simulink model "Impedance_desired"  (R2022b)
settings: Solver=VariableStepAuto  StartTime=0.0  StopTime=10.0  RelTol=1e-3
values from neighbouring files (symbols this model uses):
  Kd = diag([10,10,10,1,1,1])    [parameters.m]
  Kp = diag([190,190,190,1,1,1])    [parameters.m]
  Md = diag([0.12,0.12,0.12,0,0,0])    [parameters.m]
undefined symbols (not defined in the file or in its folder): parms
libraries: robotcorelib x1
settings Model: Creator=uzair  LastModifiedBy=uzair

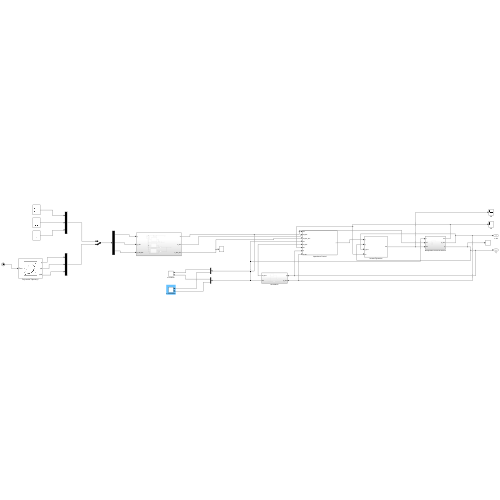
[thumbnail: Simulink's stored preview of the top-level diagram]
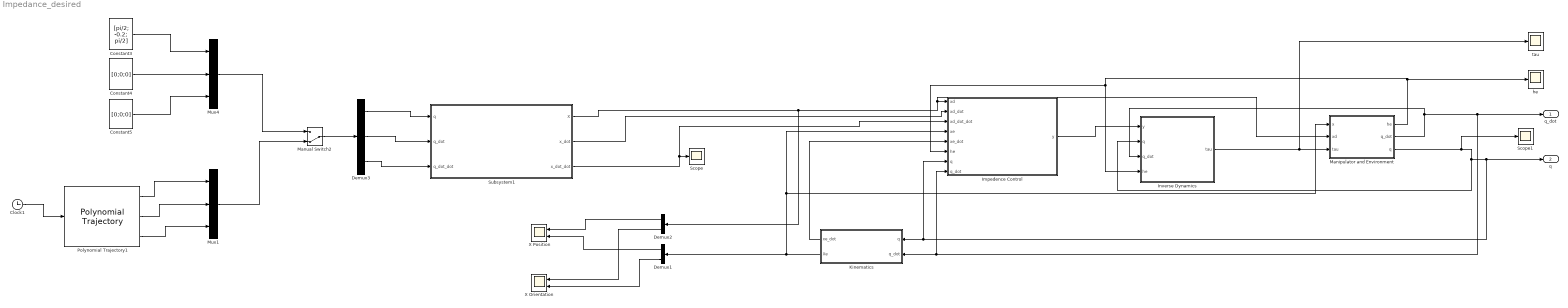
== system Impedance_desired ==
  Clock1 : Clock
  Constant3 : Constant  Value=[pi/2; -0.2; pi/2]  VectorParams1D=off
  Constant4 : Constant  Value=[0;0;0]  VectorParams1D=off
  Constant5 : Constant  Value=[0;0;0]  VectorParams1D=off
  Demux1 : Demux  Outputs=2
  Demux2 : Demux  Outputs=2
  Demux3 : Demux  Outputs=3
  Impedence Control : Subsystem
  Inverse Dynamics : Subsystem
  Kinematics : Subsystem
  Manipulator and Environment : Subsystem
  Manual Switch2 : ManualSwitch  CurrentSetting=0
  Mux1 : Mux  Inputs=3
  Mux4 : Mux  Inputs=3
  Polynomial Trajectory1 : robotcorelib/Polynomial Trajectory  WaypointSource=Internal  Waypoints=[0,0,0; 0,0,0; 0,0,0.1]  TimePoints=[ 0, 4, 9]  TimeInterval=[ 1, 4 ]  Method=Cubic Polynomial  ParameterSource=Internal  VelocityBoundaryCondition=zeros( 3,3 )  AccelerationBoundaryCondition=zeros( 3,3 )  SimulateUsing=Interpreted execution
  Scope : Scope
  Scope1 : Scope
  Subsystem1 : Subsystem
  X Orientation : Scope  NumInputPorts=2
  X Position : Scope  NumInputPorts=2
  he : Scope
  tau : Scope
  q_dot : Outport
  q : Outport  Port=2
  wires:
  Manipulator and Environment/2(q_dot) -> Inverse Dynamics/3(q_dot), Impedence Control/8(q_dot), Kinematics/2(q_dot), q_dot/1
  Manipulator and Environment/3(q) -> Scope1/1, Kinematics/1(q), Impedence Control/7(q), q/1, Inverse Dynamics/2(q)
  Inverse Dynamics/1(tau) -> tau/1, Manipulator and Environment/3(tau)
  Demux1/2 -> X Orientation/2
  Demux2/2 -> X Orientation/1
  Demux2/1 -> X Position/1
  Demux1/1 -> X Position/2
  Kinematics/2(Xe) -> Manipulator and Environment/1(x), Impedence Control/4(xe), Demux1/1
  Subsystem1/2(x_dot) -> Impedence Control/2(xd_dot)
  Subsystem1/3(x_dot_dot) -> Scope/1, Impedence Control/3(xd_dot_dot)
  Kinematics/1(xe_dot) -> Impedence Control/5(xe_dot)
  Impedence Control/1(y) -> Inverse Dynamics/1(y)
  Manipulator and Environment/1(he) -> Inverse Dynamics/4(he), Impedence Control/6(he), he/1
  Subsystem1/1(X) -> Demux2/1, Manipulator and Environment/2(xd), Impedence Control/1(xd)
  Manual Switch2/1 -> Demux3/1
  Mux4/1 -> Manual Switch2/1
  Constant4/1 -> Mux4/2
  Polynomial Trajectory1/1 -> Mux1/1
  Polynomial Trajectory1/3 -> Mux1/3
  Mux1/1 -> Manual Switch2/2
  Constant5/1 -> Mux4/3
  Demux3/1 -> Subsystem1/1(q)
  Clock1/1 -> Polynomial Trajectory1/1
  Constant3/1 -> Mux4/1
  Demux3/3 -> Subsystem1/3(q_dot_dot)
  Polynomial Trajectory1/2 -> Mux1/2
  Demux3/2 -> Subsystem1/2(q_dot)

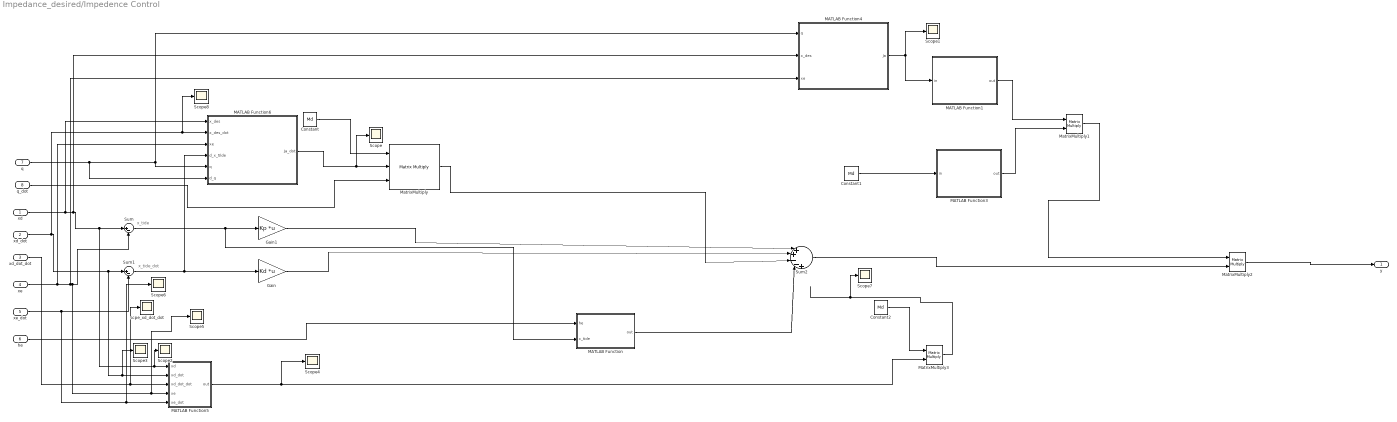
== system Impedance_desired/Impedence Control ==
  note: x_tide_dot
  note: x_tide
  xd : Inport
  xd_dot : Inport  Port=2
  xd_dot_dot : Inport  Port=3
  xe : Inport  Port=4
  xe_dot : Inport  Port=5
  he : Inport  Port=6
  q : Inport  Port=7
  q_dot : Inport  Port=8
  Constant : Constant  Value=Md  VectorParams1D=off
  Constant1 : Constant  Value=Md  VectorParams1D=off
  Constant2 : Constant  Value=Md
  Gain : Gain  Gain=Kd  Multiplication=Matrix(K*u)
  Gain1 : Gain  Gain=Kp  Multiplication=Matrix(K*u)
  MATLAB Function : MATLAB Function  TreatAsAtomicUnit=on
  MATLAB Function1 : MATLAB Function  TreatAsAtomicUnit=on
  MATLAB Function3 : MATLAB Function  TreatAsAtomicUnit=on
  MATLAB Function4 : MATLAB Function  TreatAsAtomicUnit=on
  MATLAB Function5 : MATLAB Function  TreatAsAtomicUnit=on
  MATLAB Function6 : MATLAB Function  TreatAsAtomicUnit=on
  MatrixMultiply : Product  Inputs=3  Multiplication=Matrix(*)
  MatrixMultiply1 : Product  Multiplication=Matrix(*)
  MatrixMultiply2 : Product  Multiplication=Matrix(*)
  MatrixMultiply3 : Product  Multiplication=Matrix(*)
  Scope{,1..8} (9 alike) : Scope
  Sum : Sum  Inputs=|+-
  Sum1 : Sum  Inputs=|+-
  Sum2 : Sum  Inputs=|++--+
  scpe_xd_dot_dot : Scope
  y : Outport
  wires:
  xd/1 -> MATLAB Function6/1(x_des), MATLAB Function4/2(x_des), Scope2/1, MATLAB Function5/1(xd), Sum/1
  xe/1 -> MATLAB Function6/3(xe), MATLAB Function4/3(xe), Scope5/1, MATLAB Function5/4(xe), Sum/2
  Sum/1 -> MATLAB Function/2(x_tide), Gain1/1
  xd_dot/1 -> Scope8/1, MATLAB Function6/2(x_des_dot), MATLAB Function5/2(xd_dot), Scope3/1, Sum1/1
  xe_dot/1 -> MATLAB Function5/5(xe_dot), Scope6/1, Sum1/2
  Sum1/1 -> MATLAB Function6/4(d_x_tilde), Gain/1
  Gain1/1 -> Sum2/1
  Gain/1 -> Sum2/2
  q/1 -> MATLAB Function6/6(d_q), MATLAB Function4/1(q), MATLAB Function6/5(q)
  q_dot/1 -> MatrixMultiply/3
  Constant/1 -> MatrixMultiply/1
  MATLAB Function6/1(Ja_dot) -> Scope/1, MatrixMultiply/2
  MatrixMultiply/1 -> Sum2/3
  he/1 -> MATLAB Function/1(he)
  MATLAB Function/1(out) -> Sum2/4
  MATLAB Function1/1(out) -> MatrixMultiply1/1
  MATLAB Function3/1(out) -> MatrixMultiply1/2
  MATLAB Function4/1(Ja) -> MATLAB Function1/1(in), Scope1/1
  Constant1/1 -> MATLAB Function3/1(in)
  Sum2/1 -> MatrixMultiply2/2
  MatrixMultiply1/1 -> MatrixMultiply2/1
  MatrixMultiply2/1 -> y/1
  MATLAB Function5/1(out) -> Scope4/1, MatrixMultiply3/2
  Constant2/1 -> MatrixMultiply3/1
  MatrixMultiply3/1 -> Scope7/1
  xd_dot_dot/1 -> MATLAB Function5/3(xd_dot_dot), scpe_xd_dot_dot/1

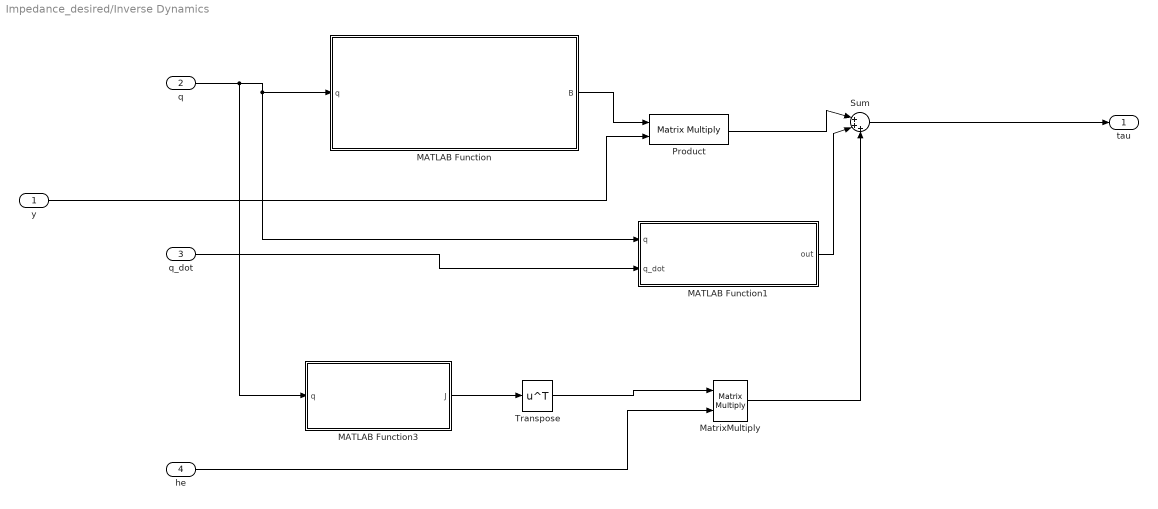
== system Impedance_desired/Inverse Dynamics ==
  y : Inport
  q : Inport  Port=2
  q_dot : Inport  Port=3
  he : Inport  Port=4
  MATLAB Function : MATLAB Function  TreatAsAtomicUnit=on
  MATLAB Function1 : MATLAB Function  TreatAsAtomicUnit=on
  MATLAB Function3 : MATLAB Function  TreatAsAtomicUnit=on
  MatrixMultiply : Product  Multiplication=Matrix(*)
  Product : Product  Multiplication=Matrix(*)
  Sum : Sum  Inputs=|+++
  Transpose : Math  Operator=transpose
  tau : Outport
  wires:
  q/1 -> MATLAB Function3/1(q), MATLAB Function1/1(q), MATLAB Function/1(q)
  MATLAB Function/1(B) -> Product/1
  y/1 -> Product/2
  q_dot/1 -> MATLAB Function1/2(q_dot)
  MATLAB Function1/1(out) -> Sum/2
  Sum/1 -> tau/1
  MATLAB Function3/1(J) -> Transpose/1
  he/1 -> MatrixMultiply/2
  Transpose/1 -> MatrixMultiply/1
  MatrixMultiply/1 -> Sum/3
  Product/1 -> Sum/1

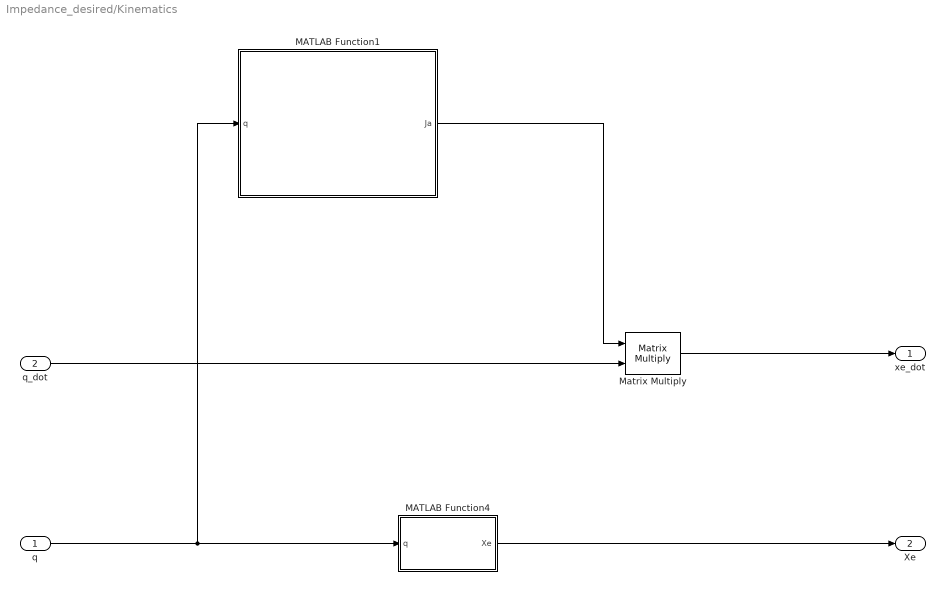
== system Impedance_desired/Kinematics ==
  q : Inport
  q_dot : Inport  Port=2
  MATLAB Function1 : MATLAB Function  TreatAsAtomicUnit=on
  MATLAB Function4 : MATLAB Function  TreatAsAtomicUnit=on
  Matrix Multiply : Product  Multiplication=Matrix(*)
  xe_dot : Outport
  Xe : Outport  Port=2
  wires:
  MATLAB Function1/1(Ja) -> Matrix Multiply/1
  q/1 -> MATLAB Function1/1(q), MATLAB Function4/1(q)
  MATLAB Function4/1(Xe) -> Xe/1
  Matrix Multiply/1 -> xe_dot/1
  q_dot/1 -> Matrix Multiply/2

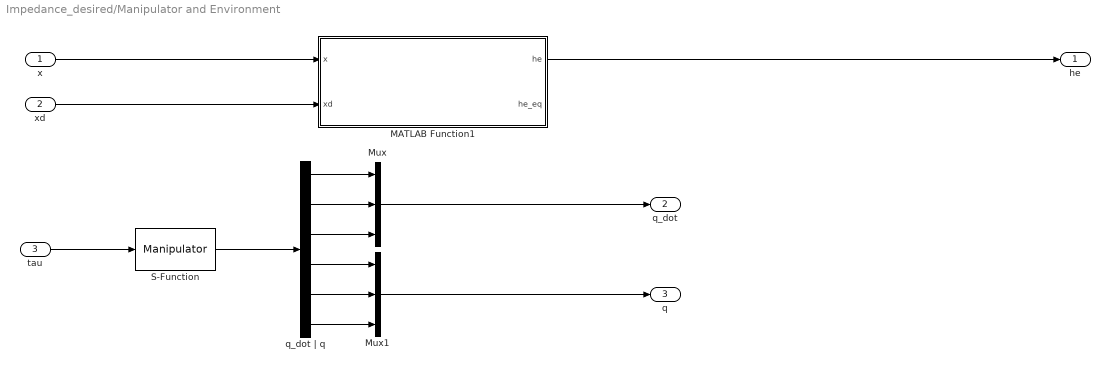
== system Impedance_desired/Manipulator and Environment ==
  x : Inport
  xd : Inport  Port=2
  tau : Inport  Port=3
  MATLAB Function1 : MATLAB Function  TreatAsAtomicUnit=on
  Mux : Mux  Inputs=3
  Mux1 : Mux  Inputs=3
  S-Function : S-Function  FunctionName=Manipulator  Parameters=params  SFunctionDeploymentMode=off  EnableBusSupport=off
  q_dot | q : Demux  Outputs=6
  he : Outport
  q_dot : Outport  Port=2
  q : Outport  Port=3
  wires:
  x/1 -> MATLAB Function1/1(x)
  xd/1 -> MATLAB Function1/2(xd)
  MATLAB Function1/1(he) -> he/1
  S-Function/1 -> q_dot | q/1
  q_dot | q/4 -> Mux1/1
  q_dot | q/1 -> Mux/1
  q_dot | q/6 -> Mux1/3
  q_dot | q/2 -> Mux/2
  q_dot | q/5 -> Mux1/2
  q_dot | q/3 -> Mux/3
  Mux/1 -> q_dot/1
  Mux1/1 -> q/1
  tau/1 -> S-Function/1

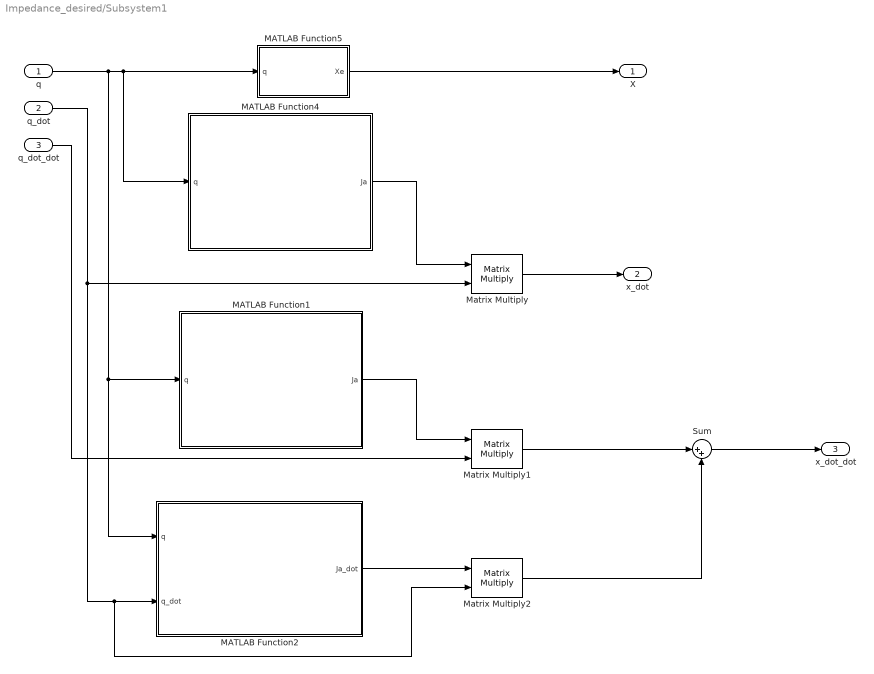
== system Impedance_desired/Subsystem1 ==
  q : Inport
  q_dot : Inport  Port=2
  q_dot_dot : Inport  Port=3
  MATLAB Function1 : MATLAB Function  TreatAsAtomicUnit=on
  MATLAB Function2 : MATLAB Function  TreatAsAtomicUnit=on
  MATLAB Function4 : MATLAB Function  TreatAsAtomicUnit=on
  MATLAB Function5 : MATLAB Function  TreatAsAtomicUnit=on
  Matrix Multiply : Product  Multiplication=Matrix(*)
  Matrix Multiply1 : Product  Multiplication=Matrix(*)
  Matrix Multiply2 : Product  Multiplication=Matrix(*)
  Sum : Sum  Inputs=|++
  X : Outport
  x_dot : Outport  Port=2
  x_dot_dot : Outport  Port=3
  wires:
  q/1 -> MATLAB Function2/1(q), MATLAB Function1/1(q), MATLAB Function4/1(q), MATLAB Function5/1(q)
  MATLAB Function5/1(Xe) -> X/1
  Matrix Multiply/1 -> x_dot/1
  q_dot/1 -> MATLAB Function2/2(q_dot), Matrix Multiply2/2, Matrix Multiply/2
  MATLAB Function4/1(Ja) -> Matrix Multiply/1
  MATLAB Function1/1(Ja) -> Matrix Multiply1/1
  q_dot_dot/1 -> Matrix Multiply1/2
  Matrix Multiply1/1 -> Sum/1
  Sum/1 -> x_dot_dot/1
  MATLAB Function2/1(Ja_dot) -> Matrix Multiply2/1
  Matrix Multiply2/1 -> Sum/2

== matlab function Impedance_desired/Inverse Dynamics/MATLAB Function3 ==
  data: q input; J output
function J = GeomatricalJacobian(q)
q1 = q(1);
q2 = q(2);
q3 = q(3);

    J = [
[                                                             0,        0,         -(4*cos(q3))/25]
[- (2*sin(q1))/5 - cos(q1)*(q2 + 3/10) - (4*cos(q3)*sin(q1))/25, -sin(q1), -(4*cos(q1)*sin(q3))/25]
[  (2*cos(q1))/5 + (4*cos(q1)*cos(q3))/25 - sin(q1)*(q2 + 3/10),  cos(q1), -(4*sin(q1)*sin(q3))/25]
[                                                             1,        0,                       0]
[                                                            0,        0,                -sin(q1)]
[                                                             0,        0,                 cos(q1)]];

end

== matlab function Impedance_desired/Impedence Control/MATLAB Function6 ==
  data: x_des input; x_des_dot input; xe input; d_x_tilde input; q input; Ja_dot output; d_q input
function Ja_dot = AnalyticalJacobian_dot(x_des, x_des_dot, xe, d_x_tilde, q, d_q)
    q1 = q(1);
    q2 = q(2);
    q3 = q(3);

    q1_dot = d_q(1);
    q2_dot = d_q(2);
    q3_dot = d_q(3);

    %1 for the Jad
    flag = 0;


    if flag == 0

    H = [[       0,         -cos(q3),        -sin(q3),                                                     -(4*sin(q3))/25]
         [ sin(q1), -cos(q1)*sin(q3), cos(q1)*cos(q3),        (2*cos(q1))/5 + (4*cos(q1)*cos(q3))/25 - sin(q1)*(q2 + 3/10)]
         [-cos(q1), -sin(q1)*sin(q3), cos(q3)*sin(q1), (2*sin(q1))/5 + cos(q1)*(q2 + 3/10) + (4*cos(q3)*sin(q1))/25 + 3/20]
         [       0,                0,               0,                                                                   1]];


        eulers = rotm2eul(H(1:3,1:3), "ZYZ");


        phi1 = eulers(1);
        phi2 = eulers(2);
        phi3 = eulers(3); %not used

        Ja_dot = [
[                                                                                                                                   0,               0,                                                 (4*q3_dot*sin(q3))/25]
[  q1_dot*sin(q1)*(q2 + 3/10) - q2_dot*cos(q1) - (4*q1_dot*cos(q1)*cos(q3))/25 - (2*q1_dot*cos(q1))/5 + (4*q3_dot*sin(q1)*sin(q3))/25, -q1_dot*cos(q1),         (4*q1_dot*sin(q1)*sin(q3))/25 - (4*q3_dot*cos(q1)*cos(q3))/25]
[- (2*q1_dot*sin(q1))/5 - q2_dot*sin(q1) - q1_dot*cos(q1)*(q2 + 3/10) - (4*q1_dot*cos(q3)*sin(q1))/25 - (4*q3_dot*cos(q1)*sin(q3))/25, -q1_dot*sin(q1),       - (4*q1_dot*cos(q1)*sin(q3))/25 - (4*q3_dot*cos(q3)*sin(q1))/25]
[                                                                                                                                   0,               0, -(q1_dot*(sin(phi2)*sin(q1) - cos(phi2)*cos(q1)*sin(phi1)))/sin(phi2)]
[                                                                                                                                   0,               0,                                             -q1_dot*cos(phi1)*cos(q1)]
[                                                                                                                                   0,               0,                                 -(q1_dot*cos(q1)*sin(phi1))/sin(phi2)]
 ];


    else
    
    J = [
        [                                                             0,        0,         -(4*cos(q3))/25]
        [- (2*sin(q1))/5 - cos(q1)*(q2 + 3/10) - (4*cos(q3)*sin(q1))/25, -sin(q1), -(4*cos(q1)*sin(q3))/25]
        [  (2*cos(q1))/5 + (4*cos(q1)*cos(q3))/25 - sin(q1)*(q2 + 3/10),  cos(q1), -(4*sin(q1)*sin(q3))/25]
        [                                                             1,        0,                       0]
        [                                                             0,        0,                -sin(q1)]
        [                                                             0,        0,                 cos(q1)]
    ];

    J_dot = [
[                                                                                                                                   0,               0,                                           (4*q3_dot*sin(q3))/25]
[  q1_dot*sin(q1)*(q2 + 3/10) - q2_dot*cos(q1) - (4*q1_dot*cos(q1)*cos(q3))/25 - (2*q1_dot*cos(q1))/5 + (4*q3_dot*sin(q1)*sin(q3))/25, -q1_dot*cos(q1),   (4*q1_dot*sin(q1)*sin(q3))/25 - (4*q3_dot*cos(q1)*cos(q3))/25]
[- (2*q1_dot*sin(q1))/5 - q2_dot*sin(q1) - q1_dot*cos(q1)*(q2 + 3/10) - (4*q1_dot*cos(q3)*sin(q1))/25 - (4*q3_dot*cos(q1)*sin(q3))/25, -q1_dot*sin(q1), - (4*q1_dot*cos(q1)*sin(q3))/25 - (4*q3_dot*cos(q3)*sin(q1))/25]
[                                                                                                                                   0,               0,                                                               0]
[                                                                                                                                   0,               0,                                                 -q1_dot*cos(q1)]
[                                                                                                                                   0,               0,                                                 -q1_dot*sin(q1)]];

     % Get euler angles from x_tilde
    x_tilde = x_des - xe;
    O_d_e = - x_tilde(4:6);
    phi = O_d_e(1);
    theta = O_d_e(2);
    
    % Get velocities along euler angles
    omega_d_e = - d_x_tilde(4:6);
    theta_dot = omega_d_e(1);
    phi_dot = omega_d_e(2);
    
    % Build rotation matrix
    Rd = eul2rotm(x_des(4:6)', 'ZYZ');
    R = [Rd', zeros(3,3); zeros(3,3), Rd'];
    
    % Get Ta and the necessary transformations
    Ta =  [1, 0, 0, 0, 0, 0;
            0, 1, 0, 0, 0, 0;
            0, 0, 1, 0, 0, 0;
            0, 0, 0, 0, -sin(phi), cos(phi) * sin(theta);
            0, 0, 0, 0, cos(phi), sin(phi) * sin(theta);
            0, 0, 0, 1, 0, cos(theta)];
    Ta_inv = pinv(Ta);
    
    % Precomputed dot inverse of Ta
    d_Ta = [[0, 0, 0, 0,                 0,                                                           0]
            [0, 0, 0, 0,                 0,                                                           0]
            [0, 0, 0, 0,                 0,                                                           0]
            [0, 0, 0, 0, -phi_dot*cos(phi), theta_dot*cos(phi)*cos(theta) - phi_dot*sin(phi)*sin(theta)]
            [0, 0, 0, 0, -phi_dot*sin(phi), phi_dot*cos(phi)*sin(theta) + theta_dot*cos(theta)*sin(phi)]
            [0, 0, 0, 0,                 0,                                       -theta_dot*sin(theta)]];
    Ta_inv_dot = pinv(d_Ta);
    
    % Build the skew symmetric matrix used to compute the derivative
    wd_d = x_des_dot(4:6);
    Swd = [   0      -wd_d(3)   wd_d(2);
              wd_d(3)       0      -wd_d(1);
             -wd_d(2)   wd_d(1)     0   ];
    

    RS = [Rd'*Swd, zeros(3,3); zeros(3,3), Rd'*Swd];
    
    Ja_dot = Ta_inv*(RS*J+R*J_dot)+Ta_inv_dot*R*J;
    end
end

== matlab function Impedance_desired/Subsystem1/MATLAB Function2 ==
  data: q input; Ja_dot output; q_dot input
function Ja_dot = AnalyticalJacobian_Dot(q, q_dot)
q1 = q(1);
q2 = q(2);
q3 = q(3);

q1_dot = q_dot(1);
q2_dot = q_dot(2);
q3_dot = q_dot(3);

H = [[       0,         -cos(q3),        -sin(q3),                                                     -(4*sin(q3))/25]
[ sin(q1), -cos(q1)*sin(q3), cos(q1)*cos(q3),        (2*cos(q1))/5 + (4*cos(q1)*cos(q3))/25 - sin(q1)*(q2 + 3/10)]
[-cos(q1), -sin(q1)*sin(q3), cos(q3)*sin(q1), (2*sin(q1))/5 + cos(q1)*(q2 + 3/10) + (4*cos(q3)*sin(q1))/25 + 3/20]
[       0,                0,               0,                                                                   1]];



eulers = rotm2eul(H(1:3,1:3), "ZYZ");


phi1 = eulers(1);
phi2 = eulers(2);
phi3 = eulers(3); %not used

Ja_dot_m = [
[                                                                                                                                   0,               0,                                                 (4*q3_dot*sin(q3))/25]
[  q1_dot*sin(q1)*(q2 + 3/10) - q2_dot*cos(q1) - (4*q1_dot*cos(q1)*cos(q3))/25 - (2*q1_dot*cos(q1))/5 + (4*q3_dot*sin(q1)*sin(q3))/25, -q1_dot*cos(q1),         (4*q1_dot*sin(q1)*sin(q3))/25 - (4*q3_dot*cos(q1)*cos(q3))/25]
[- (2*q1_dot*sin(q1))/5 - q2_dot*sin(q1) - q1_dot*cos(q1)*(q2 + 3/10) - (4*q1_dot*cos(q3)*sin(q1))/25 - (4*q3_dot*cos(q1)*sin(q3))/25, -q1_dot*sin(q1),       - (4*q1_dot*cos(q1)*sin(q3))/25 - (4*q3_dot*cos(q3)*sin(q1))/25]
[                                                                                                                                   0,               0, -(q1_dot*(sin(phi2)*sin(q1) - cos(phi2)*cos(q1)*sin(phi1)))/sin(phi2)]
[                                                                                                                                   0,               0,                                             -q1_dot*cos(phi1)*cos(q1)]
[                                                                                                                                   0,               0,                                 -(q1_dot*cos(q1)*sin(phi1))/sin(phi2)]
];

Ja_dot = Ja_dot_m;
end

== matlab function Impedance_desired/Subsystem1/MATLAB Function4 ==
  data: q input; Ja output
function Ja = AnalyticalJacobian(q)
    q1 = q(1);
    q2 = q(2);
    q3 = q(3);

    H = [[       0,         -cos(q3),        -sin(q3),                                                     -(4*sin(q3))/25]
[ sin(q1), -cos(q1)*sin(q3), cos(q1)*cos(q3),        (2*cos(q1))/5 + (4*cos(q1)*cos(q3))/25 - sin(q1)*(q2 + 3/10)]
[-cos(q1), -sin(q1)*sin(q3), cos(q3)*sin(q1), (2*sin(q1))/5 + cos(q1)*(q2 + 3/10) + (4*cos(q3)*sin(q1))/25 + 3/20]
[       0,                0,               0,                                                                   1]];


eulers = rotm2eul(H(1:3,1:3), "ZYZ");


    phi1 = eulers(1);
    phi2 = eulers(2);
    phi3 = eulers(3); %not used

Ja_m = [
[                                                             0,        0,                                             -(4*cos(q3))/25]
[- (2*sin(q1))/5 - cos(q1)*(q2 + 3/10) - (4*cos(q3)*sin(q1))/25, -sin(q1),                                     -(4*cos(q1)*sin(q3))/25]
[  (2*cos(q1))/5 + (4*cos(q1)*cos(q3))/25 - sin(q1)*(q2 + 3/10),  cos(q1),                                     -(4*sin(q1)*sin(q3))/25]
[                              -(cos(phi1)*cos(phi2))/sin(phi2),        0, (cos(q1)*sin(phi2) + cos(phi2)*sin(phi1)*sin(q1))/sin(phi2)]
[                                                    -sin(phi1),        0,                                          -cos(phi1)*sin(q1)]
[                                           cos(phi1)/sin(phi2),        0,                              -(sin(phi1)*sin(q1))/sin(phi2)]
];


    Ja = Ja_m;
end

== matlab function Impedance_desired/Subsystem1/MATLAB Function5 ==
  data: q input; Xe output
function Xe = Kinematics(q)
    q1 = q(1);
    q2 = q(2);
    q3 = q(3);
    
H = [[       0,         -cos(q3),        -sin(q3),                                                     -(4*sin(q3))/25]
[ sin(q1), -cos(q1)*sin(q3), cos(q1)*cos(q3),        (2*cos(q1))/5 + (4*cos(q1)*cos(q3))/25 - sin(q1)*(q2 + 3/10)]
[-cos(q1), -sin(q1)*sin(q3), cos(q3)*sin(q1), (2*sin(q1))/5 + cos(q1)*(q2 + 3/10) + (4*cos(q3)*sin(q1))/25 + 3/20]
[       0,                0,               0,                                                                   1]];


    eulers = rotm2eul(H(1:3,1:3), "ZYZ");

    Xe = [H(1:3,4); eulers'];
end

== matlab function Impedance_desired/Inverse Dynamics/MATLAB Function1 ==
  data: q input; out output; q_dot input; params parameter
function out = n(q, q_dot, params)
    
    m1 = params.m(1);
    m2 = params.m(2);
    m3 = params.m(3);

    q1 = q(1);
    q2 = q(2);
    q3 = q(3);

    q1_dot = q_dot(1);
    q2_dot = q_dot(2);
    q3_dot = q_dot(3);

    g = params.g;

    Fv = params.Fv;
 

    C = [[q2_dot*((3*m2)/20 + (3*m3)/10 + m2*q2 + m3*q2) - q3_dot*((4*m3*sin(2*q3))/625 + (4*m3*sin(q3))/125), q1_dot*((3*m2)/20 + (3*m3)/10 + m2*q2 + m3*q2), (2*m3*q3_dot*cos(q3)*(q2 + 3/10))/25 - q1_dot*((4*m3*sin(q3))/125 + (8*m3*cos(q3)*sin(q3))/625)]
        [                        -q1_dot*((3*m2)/20 + (3*m3)/10 + m2*q2 + m3*q2) - (2*m3*q3_dot*sin(q3))/25,                                              0,                                                                       -(2*m3*q1_dot*sin(q3))/25]
        [                      q1_dot*((4*m3*sin(2*q3))/625 + (4*m3*sin(q3))/125) + (2*m3*q2_dot*sin(q3))/25,                       (2*m3*q1_dot*sin(q3))/25,                                                                                               0]];

    G = [(g*m1*cos(q1))/5 - g*m2*((3*sin(q1))/20 - (2*cos(q1))/5 + q2*sin(q1)) + g*m3*((2*cos(q1))/5 + (2*cos(q1)*cos(q3))/25 - sin(q1)*(q2 + 3/10));
                                                                                                                        g*cos(q1)*(m2 + m3);
                                                                                                               -(2*g*m3*sin(q1)*sin(q3))/25];

    out = C*q_dot + diag(Fv)*q_dot + G;
end

== matlab function Impedance_desired/Inverse Dynamics/MATLAB Function ==
  data: q input; B output; params parameter
function B = inertiaMatrix(q, params)
    q1 = q(1); % not used in this matrix
    q2 = q(2);
    q3 = q(3);

    m1 = params.m(1);
    m2 = params.m(2);
    m3 = params.m(3);

    B = [[(195791581307*m1)/1220703125000 + (8503*m2)/40000 + (321279862557*m3)/1220703125000 + (8*m3*cos(q3)^2)/625 + (3*m2*q2)/10 + (3*m3*q2)/5 + m2*q2^2 + m3*q2^2 + (8*m3*cos(q3))/125, (2*m2)/5 + (2*m3)/5 + (2*m3*cos(q3))/25, (2*m3*sin(q3)*(q2 + 3/10))/25]
        [                                                                                                                                         (2*m2)/5 + (2*m3)/5 + (2*m3*cos(q3))/25,                                 m2 + m3,                             0]
        [                                                                                                                                                   (2*m3*sin(q3)*(q2 + 3/10))/25,                                       0,            (32637*m3)/1562500]];
end

== matlab function Impedance_desired/Subsystem1/MATLAB Function1 ==
  data: q input; Ja output
function Ja = AnalyticalJacobian(q)
    q1 = q(1);
    q2 = q(2);
    q3 = q(3);

    H = [[       0,         -cos(q3),        -sin(q3),                                                     -(4*sin(q3))/25]
[ sin(q1), -cos(q1)*sin(q3), cos(q1)*cos(q3),        (2*cos(q1))/5 + (4*cos(q1)*cos(q3))/25 - sin(q1)*(q2 + 3/10)]
[-cos(q1), -sin(q1)*sin(q3), cos(q3)*sin(q1), (2*sin(q1))/5 + cos(q1)*(q2 + 3/10) + (4*cos(q3)*sin(q1))/25 + 3/20]
[       0,                0,               0,                                                                   1]];


eulers = rotm2eul(H(1:3,1:3), "ZYZ");


    phi1 = eulers(1);
    phi2 = eulers(2);
    phi3 = eulers(3); %not used

Ja_m = [
[                                                             0,        0,                                             -(4*cos(q3))/25]
[- (2*sin(q1))/5 - cos(q1)*(q2 + 3/10) - (4*cos(q3)*sin(q1))/25, -sin(q1),                                     -(4*cos(q1)*sin(q3))/25]
[  (2*cos(q1))/5 + (4*cos(q1)*cos(q3))/25 - sin(q1)*(q2 + 3/10),  cos(q1),                                     -(4*sin(q1)*sin(q3))/25]
[                              -(cos(phi1)*cos(phi2))/sin(phi2),        0, (cos(q1)*sin(phi2) + cos(phi2)*sin(phi1)*sin(q1))/sin(phi2)]
[                                                    -sin(phi1),        0,                                          -cos(phi1)*sin(q1)]
[                                           cos(phi1)/sin(phi2),        0,                              -(sin(phi1)*sin(q1))/sin(phi2)]
];


    Ja = Ja_m;
end

== matlab function Impedance_desired/Impedence Control/MATLAB Function ==
  data: he input; out output; x_tide input
function out = he_d_e(he, x_tide)
    Rd_e = eul2rotm(x_tide(4:6)',"ZYZ");

    out = zeros(6,1);

    out(1:3) = Rd_e * he(1:3);
    out(4:6) = Rd_e  * he(4:6);
end

== matlab function Impedance_desired/Kinematics/MATLAB Function4 ==
  data: q input; Xe output
function Xe = Kinematics(q)
    q1 = q(1);
    q2 = q(2);
    q3 = q(3);
    
H = [[       0,         -cos(q3),        -sin(q3),                                                     -(4*sin(q3))/25]
[ sin(q1), -cos(q1)*sin(q3), cos(q1)*cos(q3),        (2*cos(q1))/5 + (4*cos(q1)*cos(q3))/25 - sin(q1)*(q2 + 3/10)]
[-cos(q1), -sin(q1)*sin(q3), cos(q3)*sin(q1), (2*sin(q1))/5 + cos(q1)*(q2 + 3/10) + (4*cos(q3)*sin(q1))/25 + 3/20]
[       0,                0,               0,                                                                   1]];


    eulers = rotm2eul(H(1:3,1:3), "ZYZ");

    Xe = [H(1:3,4); eulers'];
end

== matlab function Impedance_desired/Impedence Control/MATLAB Function1 ==
  data: in input; out output
function out = inv(in)
    out = pinv(in);
end

== matlab function Impedance_desired/Kinematics/MATLAB Function1 ==
  data: q input; Ja output
function Ja = AnalyticalJacobian(q)
    q1 = q(1);
    q2 = q(2);
    q3 = q(3);

    H = [[       0,         -cos(q3),        -sin(q3),                                                     -(4*sin(q3))/25]
[ sin(q1), -cos(q1)*sin(q3), cos(q1)*cos(q3),        (2*cos(q1))/5 + (4*cos(q1)*cos(q3))/25 - sin(q1)*(q2 + 3/10)]
[-cos(q1), -sin(q1)*sin(q3), cos(q3)*sin(q1), (2*sin(q1))/5 + cos(q1)*(q2 + 3/10) + (4*cos(q3)*sin(q1))/25 + 3/20]
[       0,                0,               0,                                                                   1]];


eulers = rotm2eul(H(1:3,1:3), "ZYZ");


    phi1 = eulers(1);
    phi2 = eulers(2);
    phi3 = eulers(3); %not used

Ja_m = [
[                                                             0,        0,                                             -(4*cos(q3))/25]
[- (2*sin(q1))/5 - cos(q1)*(q2 + 3/10) - (4*cos(q3)*sin(q1))/25, -sin(q1),                                     -(4*cos(q1)*sin(q3))/25]
[  (2*cos(q1))/5 + (4*cos(q1)*cos(q3))/25 - sin(q1)*(q2 + 3/10),  cos(q1),                                     -(4*sin(q1)*sin(q3))/25]
[                              -(cos(phi1)*cos(phi2))/sin(phi2),        0, (cos(q1)*sin(phi2) + cos(phi2)*sin(phi1)*sin(q1))/sin(phi2)]
[                                                    -sin(phi1),        0,                                          -cos(phi1)*sin(q1)]
[                                           cos(phi1)/sin(phi2),        0,                              -(sin(phi1)*sin(q1))/sin(phi2)]
];


    Ja = Ja_m;
end

== matlab function Impedance_desired/Manipulator and Environment/MATLAB Function1 ==
  data: x input; he output; xd input; parms parameter; Kp parameter; he_eq output
function [he,he_eq]= Environment(x, xd, parms, Kp)
    if(x(parms.plane_axis) >= parms.plane_pos(parms.plane_axis))
        xr = parms.plane_pos;

        xdes = zeros(6,1);
        xdes(parms.plane_axis) = xd(parms.plane_axis);

        xe = zeros(6,1);
        xe(parms.plane_axis) = x(parms.plane_axis);

        he = parms.Ke * (xe - xr);

        he_eq = pinv(eye(6) + parms.Ke*pinv(Kp))*parms.Ke*(xdes - xr);

    else
        he = zeros(6,1);
        he_eq = zeros(6,1);
    end
end

== matlab function Impedance_desired/Impedence Control/MATLAB Function3 ==
  data: in input; out output
function out = inv(in)
    out = pinv(in);
end

== matlab function Impedance_desired/Impedence Control/MATLAB Function4 ==
  data: q input; Ja output; x_des input; xe input
function Ja = AnalyticalJacobian(q, x_des, xe)
    
    q1 = q(1);
    q2 = q(2);
    q3 = q(3);

    %1 for the Jad
    flag = 0;


    if flag == 0

    H = [[       0,         -cos(q3),        -sin(q3),                                                     -(4*sin(q3))/25]
         [ sin(q1), -cos(q1)*sin(q3), cos(q1)*cos(q3),        (2*cos(q1))/5 + (4*cos(q1)*cos(q3))/25 - sin(q1)*(q2 + 3/10)]
         [-cos(q1), -sin(q1)*sin(q3), cos(q3)*sin(q1), (2*sin(q1))/5 + cos(q1)*(q2 + 3/10) + (4*cos(q3)*sin(q1))/25 + 3/20]
         [       0,                0,               0,                                                                   1]];


        eulers = rotm2eul(H(1:3,1:3), "ZYZ");


        phi1 = eulers(1);
        phi2 = eulers(2);
        phi3 = eulers(3); %not used

        Ja = [
               [                                                                     0,        0,                                             -(4*cos(q3))/25]
               [- (3*cos(q1))/10 - (2*sin(q1))/5 - (4*cos(q3)*sin(q1))/25 - q2*cos(q1), -sin(q1),                                     -(4*cos(q1)*sin(q3))/25]
               [  (2*cos(q1))/5 - (3*sin(q1))/10 + (4*cos(q1)*cos(q3))/25 - q2*sin(q1),  cos(q1),                                     -(4*sin(q1)*sin(q3))/25]
               [                                      -(cos(phi1)*cos(phi2))/sin(phi2),        0, (cos(q1)*sin(phi2) + cos(phi2)*sin(phi1)*sin(q1))/sin(phi2)]
               [                                                            -sin(phi1),        0,                                          -cos(phi1)*sin(q1)]
               [                                                   cos(phi1)/sin(phi2),        0,                              -(sin(phi1)*sin(q1))/sin(phi2)]];

    else
    
    J = [
        [                                                             0,        0,         -(4*cos(q3))/25]
        [- (2*sin(q1))/5 - cos(q1)*(q2 + 3/10) - (4*cos(q3)*sin(q1))/25, -sin(q1), -(4*cos(q1)*sin(q3))/25]
        [  (2*cos(q1))/5 + (4*cos(q1)*cos(q3))/25 - sin(q1)*(q2 + 3/10),  cos(q1), -(4*sin(q1)*sin(q3))/25]
        [                                                             1,        0,                       0]
        [                                                             0,        0,                -sin(q1)]
        [                                                             0,        0,                 cos(q1)]
    ];
    
    x_tilde = x_des - xe;
    Rd = eul2rotm(-x_tilde(4:6)','ZYZ');
    angles = -x_tilde(4:6);
    
    ph = -angles(1);
    th = -angles(2);
    Ta =   [1, 0, 0, 0, 0, 0;
            0, 1, 0, 0, 0, 0;
            0, 0, 1, 0, 0, 0;
            0, 0, 0, 0, -sin(ph), cos(ph) * sin(th);
            0, 0, 0, 0, cos(ph), sin(ph) * sin(th);
            0, 0, 0, 1, 0, cos(th)];
        
    Ja = pinv(Ta)*[Rd', zeros(3,3); zeros(3,3), Rd']*J;
    end
end

== matlab function Impedance_desired/Impedence Control/MATLAB Function5 ==
  data: xd input; out output; xd_dot input; xd_dot_dot input; xe input; xe_dot input
function out = b_dot(xd, xd_dot, xd_dot_dot, xe, xe_dot)

    Rd = eul2rotm(xd(4:6)', 'ZYZ');
    
    % Get x_tilde and x_tilde_dot
    x_tilde = xd - xe;
    d_x_tilde = xd_dot - xe_dot;
    
    % Get angles from x_tilde
    phi_d_e = - x_tilde(4:6); 
    phi = phi_d_e(1);
    theta = phi_d_e(2);
    theta_dot = -d_x_tilde(2);
    phi_dot = -d_x_tilde(1);
    
    % Get the transformation matrix ZYZ
    T = [0   -sin(phi)  cos(phi)*sin(theta);
         0  cos(theta)  sin(phi)*sin(theta);
         1      0                cos(theta)];
    
    % Compute T_inv_dot
    d_T = [[0,     -phi_dot*cos(phi), theta_dot*cos(phi)*cos(theta) - phi_dot*sin(phi)*sin(theta)]
            [0, -theta_dot*sin(theta), phi_dot*cos(phi)*sin(theta) + theta_dot*cos(theta)*sin(phi)]
            [0,                     0,                                       -theta_dot*sin(theta)]];
    invT = pinv(T);
    invDT = -invT*d_T*invT;
            
    % Angular velocity and linearSwd_d velocity
    wd_d = xd_dot(4:6);
    dot_wd_d = xd_dot_dot(4:6);
    
    % Skew symmetric matrix
    Swd_d = [   0      -wd_d(3)   wd_d(2);
              wd_d(3)       0      -wd_d(1);
             -wd_d(2)   wd_d(1)     0   ];
    d_Rd = Rd'*Swd_d;
    
    % o d-e and its derivatives
    oe = xe(1:3);
    od = xd(1:3);
    dot_oe = xe_dot(1:3);
    dot_od = xd_dot(1:3);
    od_dot = xd_dot(1:3);
    od_dot_dot = xd_dot_dot(1:3);
    
    
    out = [Rd'*od_dot_dot+d_Rd'*od_dot + cross(Rd'*dot_wd_d,Rd'*(od-oe)) + cross(Rd'*wd_d, Rd'*(dot_od-dot_oe));
        invDT*wd_d + invT*dot_wd_d];
end
